simulink model "potled"  (R2018a)
settings: Solver=FixedStepDiscrete  StartTime=0.0  StopTime=10.0  RelTol=1e-3
InitFcn:
  | mbd_pnt_consistency_checks(bdroot(gcs));
undefined symbols (not defined in the file): AN, B, C11, D10, J, P16, P7, P9, PCR, R16, R5, T12, T13
libraries: mbd_pnt_ec_toolbox x7
settings Model: Creator=oolonthegreat  LastModifiedBy=oolonthegreat
settings DataIOCC: ExternalInput=off  InitialState=off  SaveOutput=off  SignalLogging=off  SaveTime=off
settings OptimizationCC: DefaultParameterBehavior=Inlined  EnhancedBackFolding=on  PassReuseOutputArgsAs=Individual arguments  OptimizeBlockOrder=speed  DifferentSizesBufferReuse=on  OptimizationCustomize=off
settings DebuggingCC: InheritedTsInSrcMsg=none  SingleTaskRateTransMsg=error  ParameterTunabilityLossMsg=error  UnconnectedInputMsg=error  UnconnectedOutputMsg=error  UnconnectedLineMsg=error  UnknownTsInhSupMsg=error
settings HardwareCC: ProdBitPerPointer=32  ProdBitPerSizeT=32  ProdBitPerPtrDiffT=32  ProdLargestAtomicInteger=Long  ProdLargestAtomicFloat=Double  ProdEndianess=BigEndian  ProdWordSize=32  ProdHWDeviceType=Motorola PowerPC
settings SFSimCC: MATLABDynamicMemAlloc=off
settings RTWCC: SystemTargetFile=mbd_pnt.tlc  MakeCommand=mbd_pnt_make_rtw COPY_MDLREF_INCLUDES=0  TemplateMakefile=mbd_pnt.tmf  PostCodeGenCommand=mbd_pnt_analyzegencode(buildInfo)  Description=Model Based Design Toolbox MPC574xP Code Generation Target  GenerateReport=on  IncludeHyperlinkInReport=on  LaunchReport=on  GenerateTraceInfo=on  GenerateTraceReport=on  GenerateTraceReportSl=on  GenerateTraceReportSf=on  GenerateTraceReportEml=on
settings CodeAppCC: ForceParamTrailComments=on  IgnoreCustomStorageClasses=off  OperatorAnnotations=on  SimulinkDataObjDesc=on  SFDataObjDesc=on  InsertBlockDesc=on
settings STFCustomTargetCC: TargetLangStandard=C99 (ISO)  MultiwordLength=256  CombineOutputUpdateFcns=on  SuppressErrorStatus=on  ERTCustomFileBanners=on  SupportContinuousTime=off  SupportNonInlinedSFcns=off  RemoveResetFunc=on  MATLABClassNameForMDSCustomization=Simulink.SoftwareTarget.ERTCustomization  GRTInterface=off  SystemTargetFile=mbd_pnt.tlc
settings ERTTargetCC: TargetLangStandard=C99 (ISO)  ParMdlRefBuildCompliant=off  CompOptLevelCompliant=off  ConcurrentExecutionCompliant=off  SuppressErrorStatus=on  ModelStepFunctionPrototypeControlCompliant=off  CPPClassGenCompliant=off  UseToolchainInfoCompliant=off  InlinedParameterPlacement=NonHierarchical  ERTCustomFileTemplate=example_file_process.tlc

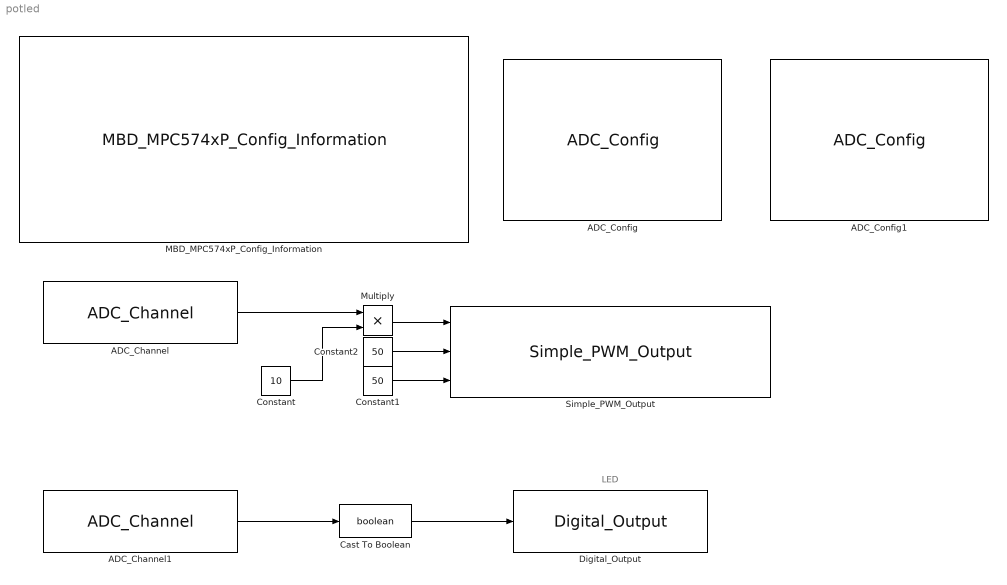
== system potled ==
  note: LED
  ADC_Channel : mbd_pnt_ec_toolbox/MPC574xP/Motor Control Blocks/ADC_Channel  adc_unit=1  adc_chan0=PCR[23] : B[7] : 43 : 51 : R5 : AN[0]  adc_chan1=PCR[76] : E[12] : 67 : 78 : T12 : AN[6]  adc_chan2=PCR[150] : J[6] : [---] : 65 : P9 : AN[1]  adc_chan3=PCR[64] : E[0] : 68 : 79 : T13 : AN[4]  simulate=off  interrupt=off  adc_mode=Normal  adc_presample=off  pcrNum=76
      settings: SourceProductName=Model Based Design Toolbox for MPC574xP
  ADC_Channel1 : mbd_pnt_ec_toolbox/MPC574xP/Motor Control Blocks/ADC_Channel  adc_unit=0  adc_chan0=PCR[24] : B[8] : 47 : 55 : P7 : AN[1]  adc_chan1=PCR[76] : E[12] : 67 : 78 : T12 : AN[6]  adc_chan2=PCR[150] : J[6] : [---] : 65 : P9 : AN[1]  adc_chan3=PCR[64] : E[0] : 68 : 79 : T13 : AN[4]  simulate=off  interrupt=off  adc_mode=Normal  adc_presample=off  pcrNum=24
      settings: SourceProductName=Model Based Design Toolbox for MPC574xP
  ADC_Config : mbd_pnt_ec_toolbox/MPC574xP/Motor Control Blocks/ADC_Config  adc_unit=1  adc_ctu=off  adc_owr=on  adc_wls=0: Left  adc_clk=on  adc_ack=on  adc_edglev=0: Edge  adc_trgen=off  adc_edge=off  adc_ctr0_samp=22  adc_ctr1_samp=11  adc_pscr_preval0=00: AGND_3V  adc_pscr_preconv=off  adc_calbist_admode=110: 12-bit operating mode (high accuracy)  adc_calbist_tsamp=00: 22 cycles of ADC clk  adc_calbist_nrsmpl=01: 32 samples  adc_calbist_avgen=on
      settings: SourceProductName=Model Based Design Toolbox for MPC574xP
  ADC_Config1 : mbd_pnt_ec_toolbox/MPC574xP/Motor Control Blocks/ADC_Config  adc_unit=0  adc_ctu=off  adc_owr=on  adc_wls=0: Left  adc_clk=on  adc_ack=on  adc_edglev=0: Edge  adc_trgen=off  adc_edge=off  adc_ctr0_samp=22  adc_ctr1_samp=11  adc_pscr_preval0=00: AGND_3V  adc_pscr_preconv=off  adc_calbist_admode=110: 12-bit operating mode (high accuracy)  adc_calbist_tsamp=00: 22 cycles of ADC clk  adc_calbist_nrsmpl=01: 32 samples  adc_calbist_avgen=on
      settings: SourceProductName=Model Based Design Toolbox for MPC574xP
  Cast To Boolean : DataTypeConversion  OutDataTypeStr=boolean
  Constant : Constant  Value=10  OutDataTypeStr=uint32
  Constant1 : Constant  Value=50  OutDataTypeStr=uint32
  Constant2 : Constant  Value=50  OutDataTypeStr=uint32
  Digital_Output : mbd_pnt_ec_toolbox/MPC574xP/Peripheral Interface Blocks/Digital_Output  gpio_outputs="43   : C11 :  [80]   : [97]   : [P16]"  pinNum=[80]  pcrNum=43
      settings: SourceProductName=Model Based Design Toolbox for MPC574xP
  MBD_MPC574xP_Config_Information : mbd_pnt_ec_toolbox/MPC574xP/MBD_MPC574xP_Config_Information  disp_str=|  config_params=[]
      | System Clock : 200 MHz
      | Target : MPC5744P
      | Package : 144LQFP
      | XTAL Freq : 40 MHz
      | Compiler : S32 Design Studio
      | Target Type : FLASH
      | Global Interrupt Priority : 8
      | System Tick Interrupt Priority : 12
      | Freemaster : Serial1 (115200 Kbits)
      | Download Code after build : (COM5,115200)
      settings: SourceProductName=Model Based Design Toolbox for MPC574xP
  Multiply : Product  OutDataTypeStr=uint32
  Simple_PWM_Output : mbd_pnt_ec_toolbox/MPC574xP/Motor Control Blocks/Simple_PWM_Output  pwmModule=0  pwmMod=0  SubModule=0  subMod=0  InitFreq=2000  resolution=1 %  resValue=1  InitDutyA=50  InitDutyB=50  align=center aligned  PhaseShift_A=0  PhaseShift_B=0  Phase_A=0  Phase_B=0  centered=1  doubleSw=off  DoubleS=0  debugSw=off  debug_mode=0  pin0_A0="58: D10 : [76]   : [93]   : [R16]"  pin0_B0=None  pin0_X0=None  pin0_A1=None  pin0_B1=None  pin0_X1=None  pin0_A2=None  pin0_B2=None  pin0_X2=None  pin0_A3=None  pin0_B3=None  pin0_X3=None  pin1_A0=None  pin1_B0=None  pin1_X0=None  pin1_A1=None  pin1_B1=None  pin1_X1=None  pin1_A2=None  pin1_B2=None  pin1_X2=None  pin1_A3=None  pin1_B3=None  pin1_X3=None  pin2_A0=None  pin2_B0=None  pin2_X0=None  pin2_A1=None  pin2_B1=None  pin2_X1=None  pin2_A2=None  pin2_B2=None  pin2_X2=None  pin2_A3=None  pin2_B3=None  pin2_X3=None  pcrNumA=58  pcrNumB=255  pcrNumX=255  polA=off  polB=off  polX=off  octrl=0  syncFrom0=off  masterSync=0  outVal0=off  outVal1=off  outVal2=off  outVal3=off  outVal4=off  outVal5=off  outTrig=0
      settings: SourceProductName=Model Based Design Toolbox for MPC574xP
  wires:
  Constant2/1 -> Simple_PWM_Output/2
  Constant1/1 -> Simple_PWM_Output/3
  Multiply/1 -> Simple_PWM_Output/1
  Constant/1 -> Multiply/2
  ADC_Channel/1 -> Multiply/1
  Cast To Boolean/1 -> Digital_Output/1
  ADC_Channel1/1 -> Cast To Boolean/1
